simulink model "Read_DTC_Fusion_cabin_sensor"  (R2019b)
settings: Solver=VariableStepAuto  StartTime=0.0  StopTime=inf  RelTol=1e-3
undefined symbols (not defined in the file): canChannel
libraries: canlib x3, canmsglib x3
settings Model: Creator=cordunoalbarran  LastModifiedBy=cordunoalbarran
settings DataIOCC: ReturnWorkspaceOutputs=off
settings DebuggingCC: ArithmeticOperatorsInVariantConditions=warning
settings SFSimCC: CustomCodeUndefinedFunction=UseInterfaceOnly

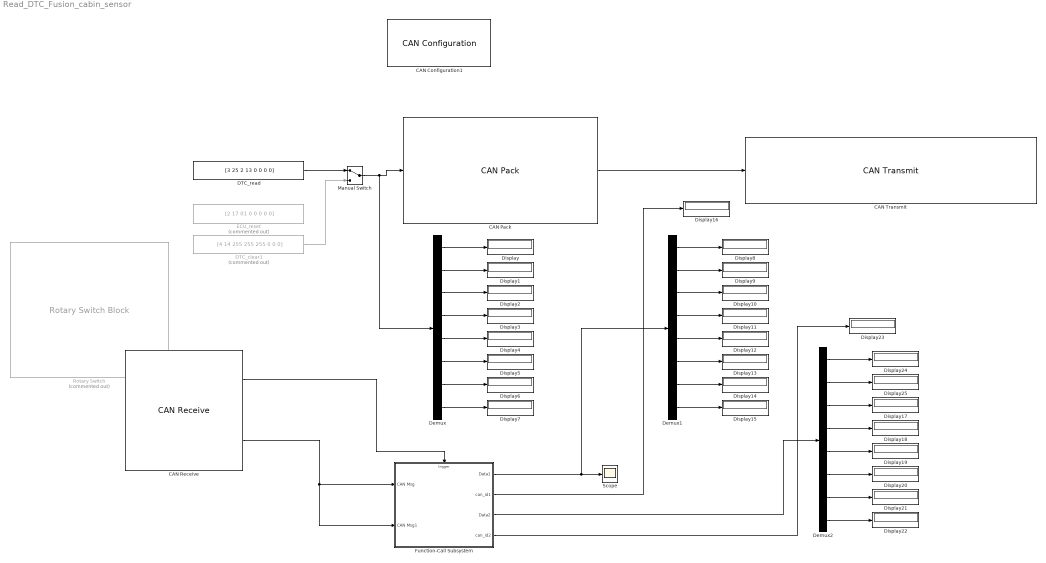
== system Read_DTC_Fusion_cabin_sensor ==
  CAN Configuration1 : canlib/CAN Configuration  BlockHandle=3.0001  Device=PEAK-System PCAN-USB (PCAN_USBBUS1)  DeviceMenu=PEAK-System PCAN-USB (PCAN_USBBUS1)  ObjConstructor=canChannel('PEAK-System', 'PCAN_USBBUS1')  BusSpeed=500000  EnableBitParameters=off  AckMode=Normal
      settings: SourceProductName=Vehicle Network Toolbox  SourceProductBaseCode=VN
  CAN Pack : canmsglib/CAN Pack  CANdbFile=C:\Users\cordunoalbarran\Documents\GUv0 Design Docs\CAN\ccan_diagnostic.dbc  MsgList=D_RQ_FUSION_CC  MsgName=D_RQ_FUSION_CC  MsgIDType=Standard (11-bit identifier)  MsgIdentifier=1959  MsgLength=8  Remote=off  ApplyMinMax=off  BusOutput=off  SignalInfo={'D_RQ_FUSION_CC','56','64','BE','unsigned','Standard','0','1','0','-Inf','Inf'}
      settings: SourceProductName=Simulink Real-Time  SourceProductBaseCode=XP  DataFormat=raw data
  CAN Receive : canlib/CAN Receive  BlockHandle=5.0001  Device=PEAK-System PCAN-USB (PCAN_USBBUS1)  DeviceMenu=PEAK-System PCAN-USB (PCAN_USBBUS1)  ObjConstructor=canChannel('PEAK-System', 'PCAN_USBBUS1')  EnableStandardIDsFilter=off  StdIDsCombo=Allow all  StandardIDs=0  EnableExtendedIDsFilter=off  ExtIDsCombo=Allow all  ExtendedIDs=0  SampleTime=0.01  MsgsPerTimestep=all  InternalFilterUpdateStatus=on  BusOutput=off
      settings: SourceProductName=Vehicle Network Toolbox  SourceProductBaseCode=VN
  CAN Transmit : canlib/CAN Transmit  BlockHandle=6.0001  Device=PEAK-System PCAN-USB (PCAN_USBBUS1)  DeviceMenu=PEAK-System PCAN-USB (PCAN_USBBUS1)  ObjConstructor=canChannel('PEAK-System', 'PCAN_USBBUS1')  EnablePeriodicTransmit=on  MessagePeriod=4
      settings: SourceProductName=Vehicle Network Toolbox  SourceProductBaseCode=VN
  DTC_clear1 : Constant  Commented=on  Value=[4 14 255 255 255 0 0 0]  OutDataTypeStr=uint8  SampleTime=0.01
  DTC_read : Constant  Value=[3 25 2 13 0 0 0 0]  OutDataTypeStr=uint8  SampleTime=0.01
  Demux : Demux  Outputs=8
  Demux1 : Demux  Outputs=8
  Demux2 : Demux  Outputs=8
  Display{,1..25} (26 alike) : Display
  ECU_reset : Constant  Commented=on  Value=[2 17 01 0 0 0 0 0]  OutDataTypeStr=uint8  SampleTime=0.01
  Function-Call Subsystem : Subsystem  TreatAsAtomicUnit=on
  Manual Switch : ManualSwitch
  Rotary Switch : RotarySwitchBlock  Commented=on
      settings: Values={{'Off', 'DTC_read', 'DTC_clear'}, [0 1 2]}
  Scope : Scope
  wires:
  CAN Pack/1 -> CAN Transmit/1
  CAN Receive/2 -> Function-Call Subsystem/2(CAN Msg1), Function-Call Subsystem/1(CAN Msg)
  CAN Receive/1 -> Function-Call Subsystem/Trigger
  Manual Switch/1 -> Demux/1, CAN Pack/1
  DTC_read/1 -> Manual Switch/1
  Demux/1 -> Display/1
  Demux/2 -> Display1/1
  Demux/3 -> Display2/1
  Demux/4 -> Display3/1
  Demux/5 -> Display4/1
  Demux/6 -> Display5/1
  Demux/7 -> Display6/1
  Demux/8 -> Display7/1
  Demux1/8 -> Display15/1
  Demux1/7 -> Display14/1
  Demux1/6 -> Display13/1
  Demux1/5 -> Display12/1
  Demux1/4 -> Display11/1
  Demux1/3 -> Display10/1
  Demux1/2 -> Display9/1
  Demux1/1 -> Display8/1
  Function-Call Subsystem/1(Data1) -> Demux1/1, Scope/1
  Function-Call Subsystem/2(can_id1) -> Display16/1
  Demux2/3 -> Display17/1
  Demux2/2 -> Display25/1
  Demux2/1 -> Display24/1
  Demux2/6 -> Display20/1
  Demux2/8 -> Display22/1
  Demux2/7 -> Display21/1
  Demux2/5 -> Display19/1
  Demux2/4 -> Display18/1
  Function-Call Subsystem/3(Data2) -> Demux2/1
  Function-Call Subsystem/4(can_id2) -> Display23/1
  DTC_clear1/1 -> Manual Switch/2

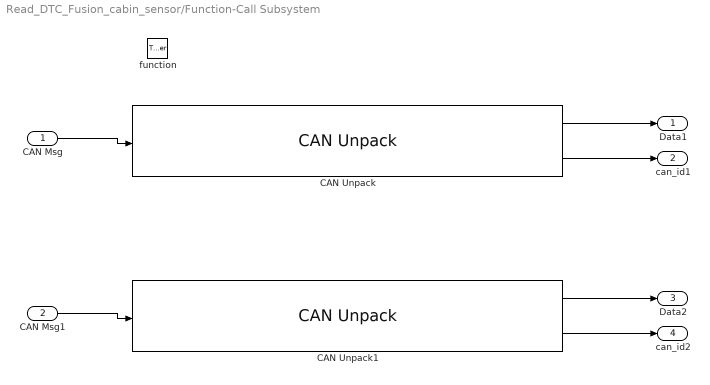
== system Read_DTC_Fusion_cabin_sensor/Function-Call Subsystem ==
  CAN Msg : Inport
  CAN Msg1 : Inport  Port=2
  function : TriggerPort  TriggerType=function-call  VariantControl=Variant
  CAN Unpack : canmsglib/CAN Unpack  CANdbFile=C:\Users\cordunoalbarran\Documents\GUv0 Design Docs\CAN\ccan_diagnostic.dbc  MsgList=D_RS_FUSION_CC  MsgName=D_RS_FUSION_CC  MsgIDType=Standard (11-bit identifier)  MsgIdentifier=1967  MsgLength=8  SignalInfo={ 'D_RS_FUSION_CC', '56', '64', 'BE', 'unsigned', 'Standard', '0', '1', '0', '-Inf', 'Inf' }  IDPort=on  TimestampPort=off  ErrorPort=off  RemotePort=off  LengthPort=off  StatusPort=off  ApplyMinMax=off
      settings: SourceProductName=Simulink Real-Time  SourceProductBaseCode=XP  DataFormat=raw data
  CAN Unpack1 : canmsglib/CAN Unpack  CANdbFile=C:\Users\cordunoalbarran\Documents\GUv0 Design Docs\CAN\ccan_diagnostic.dbc  MsgList=D_RQ_FUSION_CC  MsgName=D_RQ_FUSION_CC  MsgIDType=Standard (11-bit identifier)  MsgIdentifier=1959  MsgLength=8  SignalInfo={ 'D_RS_FUSION_CC', '56', '64', 'BE', 'unsigned', 'Standard', '0', '1', '0', '-Inf', 'Inf' }  IDPort=on  TimestampPort=off  ErrorPort=off  RemotePort=off  LengthPort=off  StatusPort=off  ApplyMinMax=off
      settings: SourceProductName=Simulink Real-Time  SourceProductBaseCode=XP  DataFormat=raw data
  Data1 : Outport  VectorParamsAs1DForOutWhenUnconnected=off
  can_id1 : Outport  Port=2
  Data2 : Outport  Port=3  VectorParamsAs1DForOutWhenUnconnected=off
  can_id2 : Outport  Port=4
  wires:
  CAN Msg/1 -> CAN Unpack/1
  CAN Unpack/1 -> Data1/1
  CAN Unpack/2 -> can_id1/1
  CAN Unpack1/1 -> Data2/1
  CAN Msg1/1 -> CAN Unpack1/1
  CAN Unpack1/2 -> can_id2/1
